simulink model "mpc_v2"  (Simulink 8.4)
settings: Solver=FixedStepDiscrete  StartTime=0  StopTime=inf  RelTol=1e-3
PreLoadFcn:
  | openecu_make_rtw_hook('model_load', 'mpc_v2')
PostLoadFcn:
  | openecu_make_rtw_hook('model_loaded', 'mpc_v2')
InitFcn:
  | openecu_make_rtw_hook('model_init',   'mpc_v2')
undefined symbols (not defined in the file or in its folder): Fbrake, Grade, h, km, N, PRND, Torque_Req, v_ref, Velocity
libraries: pcx x4, simulink x1, mpclib x1, pcp_CCP_Configuration x1, prtw x1, put x1
settings Model: Creator=jtough  LastModifiedBy=Administrator
settings ConfigSet: Description=|
  | OpenECU configuration set for code generation under RTW (RSIM).
  | --
  | OpenECU RTW (RSIM) support is deprecated, please use the OpenECU RTW (RTMODEL) configuration set.
settings SolverCC: PositivePriorityOrder=on
settings OptimizationCC: InlineParams=on  InlineInvariantSignals=on  EnhancedBackFolding=on  FoldNonRolledExpr=off
settings DebuggingCC: SaveWithParameterizedLinksMsg=none  SignalResolutionControl=TryResolveAllWithWarning  SolverPrmCheckMsg=none  MultiTaskDSMMsg=warning  MultiTaskCondExecSysMsg=none  MultiTaskRateTransMsg=warning  CheckMatrixSingularityMsg=warning  VectorMatrixConversionMsg=warning  SignalLabelMismatchMsg=warning
settings HardwareCC: ProdLargestAtomicInteger=Long  ProdLargestAtomicFloat=Double  ProdIntDivRoundTo=Zero  ProdEndianess=BigEndian  ProdHWDeviceType=Freescale->32-bit PowerPC  TargetLargestAtomicInteger=Long  TargetLargestAtomicFloat=Double  TargetIntDivRoundTo=Zero  TargetEndianess=BigEndian  TargetHWDeviceType=Freescale->32-bit PowerPC  ProdEqTarget=off
settings RTWCC: SystemTargetFile=openecu.tlc  TemplateMakefile=openecu_r2014b_64.tmf  Description=OpenECU Platform Target (GRT, RSIM based)  RetainRTWFile=on  ProcessScript=openecu_make_rtw_hook  IncludeERTFirstTime=on
settings STFCustomTargetCC: TargetLibSuffix=.a  ModelReferenceCompliant=off  GeneratePreprocessorConditionals=Disable all  MATLABClassNameForMDSCustomization=Simulink.SoftwareTarget.TargetSpecificTriggerConfigurationBase  SystemTargetFile=openecu.tlc
settings RSimTargetCC: TargetLibSuffix=.a  ERTMultiwordTypeDef=System defined  ERTMultiwordLength=256  ModelReferenceCompliant=off  ParMdlRefBuildCompliant=off  CompOptLevelCompliant=off  ConcurrentExecutionCompliant=off  MatFileLogging=off  EnableShiftOperators=on
settings EnumStrPairs: String=prefix_name

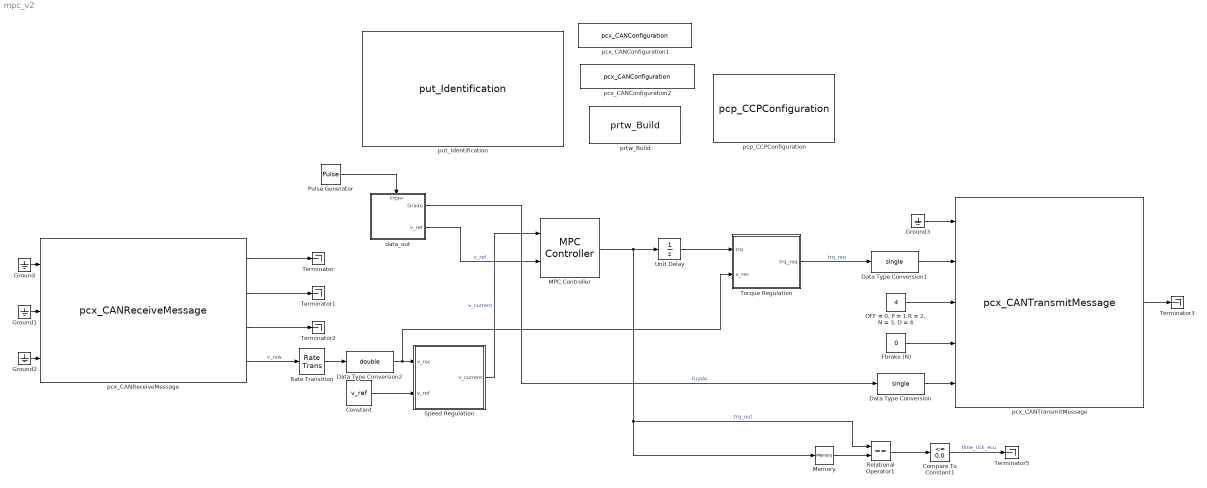
== system mpc_v2 ==
  Compare To Constant1 : simulink/Logic and Bit Operations/Compare To Constant  relop=<=  const=0.0  OutDataTypeStr=boolean
  Constant : Constant  Value=v_ref
  Data Type Conversion : DataTypeConversion  OutDataTypeStr=single  RndMeth=Nearest
  Data Type Conversion1 : DataTypeConversion  OutDataTypeStr=single  RndMeth=Nearest
  Data Type Conversion2 : DataTypeConversion  OutDataTypeStr=double  RndMeth=Nearest
  Fbrake (N) : Constant  Value=0  OutDataTypeStr=single
  Ground{,1..3} (4 alike) : Ground
  MPC Controller : mpclib/MPC Controller  SCDEnableBlockLinearizationSpecification=on  mpcobj=mpc_controller_v1  is_multiple=0  enable_value=0  n_mv=1  n_mo=1  n_md=0  n_ts=0.1  is_designfromscratch=0  return_u0=off  ref_from_ws=off  ref_signal_name=[]  ref_preview=off  md_from_ws=off  md_signal_name=[]  md_preview=off  from_project=off  project_file=MPCtask.mat  md_inport=off  mv_inport=off  cost_outport=off  return_sequence=off  return_qpstatus=off  return_state=off  state_inport=off  lims_inport=off  ywt_inport=off  uwt_inport=off  duwt_inport=off  rhoeps_inport=off  uref_inport=off  BlockDataType=double  SampleTimeInherited=off  switch_inport=off
  Memory : Memory
  "OFF = 0, P = 1 R = 2, N = 3, D = 4" : Constant  Value=4  OutDataTypeStr=single
  Pulse Generator : DiscretePulseGenerator  PulseType=Time based  Period=1  PulseWidth=10
  Rate Transition : RateTransition  OutPortSampleTime=0.1
  Relational Operator1 : RelationalOperator  Operator===  OutDataTypeStr=boolean
  Speed Regulation : MATLAB Function  TreatAsAtomicUnit=on
  Terminator{,1..3,5} (5 alike) : Terminator
  Torque Regulation : MATLAB Function  TreatAsAtomicUnit=on
  Unit Delay : UnitDelay  SampleTime=-1
  data_out : Subsystem
  pcp_CCPConfiguration : pcp_CCP_Configuration/pcp_CCPConfiguration  pcpl_rx_msgid=1785  pcpl_tx_msgid=1784  pcpl_station_id=0  bus_id=CAN 0 (pin A28+A43)  pcpl_ccpenabled=on  pcpl_rx_ext_id=off  pcpl_tx_ext_id=off  pcpl_caltool=Generic
  pcx_CANConfiguration1 : pcx/pcx_CANConfiguration  bit_rate=1000 kBps  bus_id=CAN 0 (pin A28+A43)
  pcx_CANConfiguration2 : pcx/pcx_CANConfiguration  bit_rate=1000 kBps  bus_id=CAN 1 (pin A29+A44)
  pcx_CANReceiveMessage : pcx/pcx_CANReceiveMessage  pcxl_msg_id=257  pcxl_msg_length=8  pcxl_field_start_pos=[0]  pcxl_field_width=[8]  pcxl_field_is_signed=[0]  pcxl_type_codes=[0]  pcxl_field_mnemonics=Velocity(km/h)  bus_id=CAN 0 (pin A28+A43)  pcxl_sample_time=0.01  pcxl_use_extended_ids=off  pcxl_provide_timestamp=off  pcxl_provide_sim_inputs=off
  pcx_CANTransmitMessage : pcx/pcx_CANTransmitMessage  pcxl_msg_id=1025  pcxl_msg_length=8  pcxl_field_start_pos=[0,8,16,24]  pcxl_field_width=[8,8,8,8]  pcxl_field_is_signed=[0,0,0,0]  pcxl_type_codes=[0,0,0,0]  pcxl_field_mnemonics=Torque_Req(N.m), PRND, Fbrake(N), Grade(%)  bus_id=CAN 0 (pin A28+A43)  pcxl_use_extended_ids=off  pcxl_provide_status=off  pcxl_provide_sim_outputs=off
  prtw_Build : prtw/prtw_Build
  put_Identification : put/put_Identification  put_id_marque=M250  dummy_marque_00=01T-068883-000  dummy_marque_01=01T-068432-000  dummy_marque_02=01T-068696-000  dummy_marque_03=01T-068276-000  dummy_marque_04=01T-068144-000  dummy_marque_05=01T-068148-000  dummy_marque_06=01T-068787-000  dummy_marque_07=01T-063512-000  dummy_marque_08=01T-068148-000  dummy_marque_09=01T-068408-000  dummy_marque_10=01T-063522-000  put_id_part_number=01T-068276-000  put_id_num_marques=7  put_id_max_marques=11  put_id_issue_number=3  put_id_min_issue_num=2  put_id_naming=Generic pin naming  put_id_name=MPC Design  put_id_description=(none)  put_id_major_ver_str=1  put_id_major_ver_num=1  put_id_minor_ver_str=0  put_id_minor_ver_num=0  put_id_subminor_ver_str=0  put_id_subminor_ver_num=0  put_id_copyright=(none)  put_id_target=Unused  put_id_target_type=M250  put_id_subtype=000  put_id_family=Unused  put_id_variant=Unused  put_id_A450_variant=0  put_id_G400_variant=0  put_id_G800_variant=0  put_id_G850_variant=Unused  put_id_M001_variant=0  put_id_M250_variant=Unused  put_id_M460_variant=Unused  put_id_M461_variant=Unused  put_id_U082_variant=Unused  put_id_U82_variant=Unused
  wires:
  pcx_CANReceiveMessage/2 -> Terminator1/1
  pcx_CANReceiveMessage/1 -> Terminator/1
  pcx_CANReceiveMessage/3 -> Terminator2/1
  Ground2/1 -> pcx_CANReceiveMessage/3
  Ground1/1 -> pcx_CANReceiveMessage/2
  Ground/1 -> pcx_CANReceiveMessage/1
  pcx_CANTransmitMessage/1 -> Terminator3/1
  "OFF = 0, P = 1 R = 2, N = 3, D = 4"/1 -> pcx_CANTransmitMessage/3
  Fbrake (N)/1 -> pcx_CANTransmitMessage/4
  Ground3/1 -> pcx_CANTransmitMessage/1
  Data Type Conversion/1 -> pcx_CANTransmitMessage/5
  Pulse Generator/1 -> data_out/Trigger
  data_out/2(v_ref) -> MPC Controller/2  "v_ref"
  data_out/1(Grade) -> Data Type Conversion/1  "Grade"
  MPC Controller/1 -> Memory/1, Relational Operator1/1, Unit Delay/1  "trq_out"
  Constant/1 -> Speed Regulation/2(v_ref)
  Speed Regulation/1(v_current) -> MPC Controller/1  "v_current"
  Unit Delay/1 -> Torque Regulation/1(trq)
  Torque Regulation/1(trq_req) -> Data Type Conversion1/1  "trq_req"
  Data Type Conversion1/1 -> pcx_CANTransmitMessage/2
  pcx_CANReceiveMessage/4 -> Rate Transition/1  "v_raw"
  Data Type Conversion2/1 -> Speed Regulation/1(v_rec), Torque Regulation/2(v_rec)
  Memory/1 -> Relational Operator1/2
  Relational Operator1/1 -> Compare To Constant1/1
  Compare To Constant1/1 -> Terminator5/1  "time_tick_ecu"
  Rate Transition/1 -> Data Type Conversion2/1

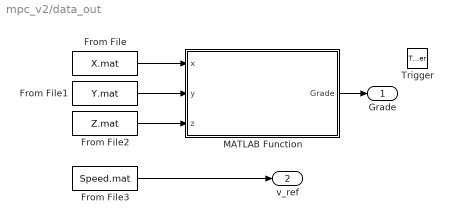
== system mpc_v2/data_out ==
  Trigger : TriggerPort  PortDimensions=1
  From File : FromFile  FileName=X.mat
  From File1 : FromFile  FileName=Y.mat
  From File2 : FromFile  FileName=Z.mat
  From File3 : FromFile  FileName=Speed.mat
  MATLAB Function : MATLAB Function  TreatAsAtomicUnit=on
  Grade : Outport
  v_ref : Outport  Port=2
  wires:
  From File2/1 -> MATLAB Function/3(z)
  From File1/1 -> MATLAB Function/2(y)
  From File/1 -> MATLAB Function/1(x)
  MATLAB Function/1(Grade) -> Grade/1
  From File3/1 -> v_ref/1

== matlab function Speed Regulation ==
  data: v_rec input double; v_current output double; v_ref input double
function v_current = fcn(v_rec,v_ref)

if v_rec < 51 && v_rec >= 1
    v_current = v_rec;
else
    v_current = v_ref;
end

== matlab function data_out/MATLAB Function ==
  data: x input double; y input double; z input double; Grade output double
function Grade = convert_to_grade(x,y,z)

state_init = 0;
state = sqrt((x^2)+(y^2)+(z^2));
state = state + state_init;
r = sqrt((x^2)+(y^2));
alpha = acos(r / state);
Grade = alpha*100;

== matlab function Torque Regulation ==
  data: trq input double; trq_req output double; v_rec input double
function trq_req = fcn(trq,v_rec)

if v_rec < 51 && v_rec >= 1
    if trq > 290
        trq_req = 290;
    elseif trq < -290
        trq_req = -290;
    else
        trq_req = trq;
    end
else
    trq_req = 60;
end
